simulink model "F_sim"  (R2017a)
settings: Solver=ode45  StartTime=0.0  StopTime=10000  MaxStep=.1  RelTol=1e-3  EnableMultiTasking=on
InitFcn:
  | addpath ./..
  | % E_param.m
undefined symbols (not defined in the file or in its folder): F_animation
libraries: simulink x4
settings Model: Creator=beard  LastModifiedBy=Mat Haskell
settings DataIOCC: LimitDataPoints=on  SaveFormat=Array  SignalLoggingSaveFormat=ModelDataLogs
settings OptimizationCC: ExpressionDepthLimit=2147483647  InitFltsAndDblsToZero=on  LifeSpan=inf
settings DebuggingCC: UnderspecifiedInitializationDetection=Classic  MergeDetectMultiDrivingBlocksExec=none  SolverPrmCheckMsg=warning  FcnCallInpInsideContextMsg=warning  StateNameClashWarn=warning  SFUnexpectedBacktrackingDiag=warning  SFNoUnconditionalDefaultTransitionDiag=warning  SFExecutionAtInitializationDiag=none
settings HardwareCC: ProdBitPerPointer=32  ProdBitPerSizeT=32  ProdBitPerPtrDiffT=32  ProdLargestAtomicFloat=None  ProdIntDivRoundTo=Undefined  ProdEndianess=Unspecified  ProdWordSize=32  ProdHWDeviceType=32-bit Generic
settings ModelReferenceCC: PropagateSignalLabelsOutOfModel=off
settings GRTTargetCC: TargetLangStandard=C89/C90 (ANSI)  GeneratePreprocessorConditionals=Disable all  CombineOutputUpdateFcns=off  GRTInterface=on
settings ConfigComp: CovMetricSettings=dw  CovHtmlReporting=on  CovSaveCumulativeToWorkspaceVar=on  CovSaveSingleToWorkspaceVar=on  CovExternalEMLEnable=off

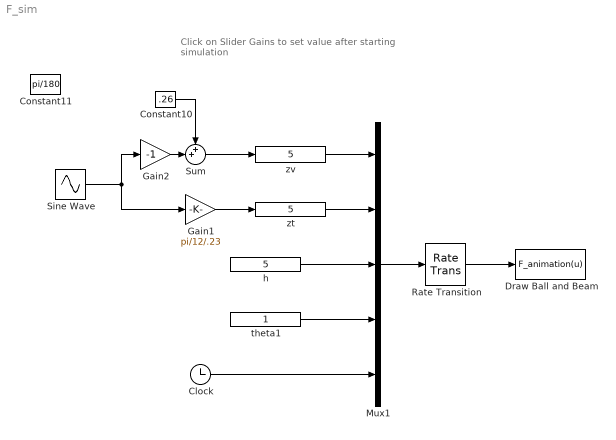
== system F_sim ==
  note: Click on Slider Gains to set value
      | after starting simulation
  Clock : Clock
  Constant10 : Constant  Value=.26
  Constant11 : Constant  Value=pi/180
  Draw Ball and Beam : MATLABFcn  InitFcn=|  MATLABFcn=F_animation(u)  OutputDimensions=0
      | clear;clc
      | F_param
  Gain1 : Gain  Gain=pi/12/.23
  Gain2 : Gain  Gain=-1
  Mux1 : Mux  Inputs=5
  Rate Transition : RateTransition  OutPortSampleTime=P.t_plot
  Sine Wave : Sin  Amplitude=.23  SampleTime=0
  Sum : Sum  Inputs=++|
  h : simulink/Math Operations/Slider Gain  gain=5  low=-90  high=90
  theta1 : simulink/Math Operations/Slider Gain  gain=1  low=-180  high=180
  zt : simulink/Math Operations/Slider Gain  gain=5  low=2  high=8
  zv : simulink/Math Operations/Slider Gain  gain=5  low=2  high=8
  wires:
  zv/1 -> Mux1/1
  Clock/1 -> Mux1/5
  zt/1 -> Mux1/2
  h/1 -> Mux1/3
  theta1/1 -> Mux1/4
  Mux1/1 -> Rate Transition/1
  Rate Transition/1 -> Draw Ball and Beam/1
  Sine Wave/1 -> Gain2/1, Gain1/1
  Gain1/1 -> zt/1
  Constant10/1 -> Sum/1
  Sum/1 -> zv/1
  Gain2/1 -> Sum/2
